simulink model "vehiclemodel"  (R2019a)
settings: Solver=VariableStepAuto  StartTime=0.0  StopTime=10.0  RelTol=1e-3
libraries: simulink x2, autolibshared x1
settings Model: Creator=L  LastModifiedBy=L

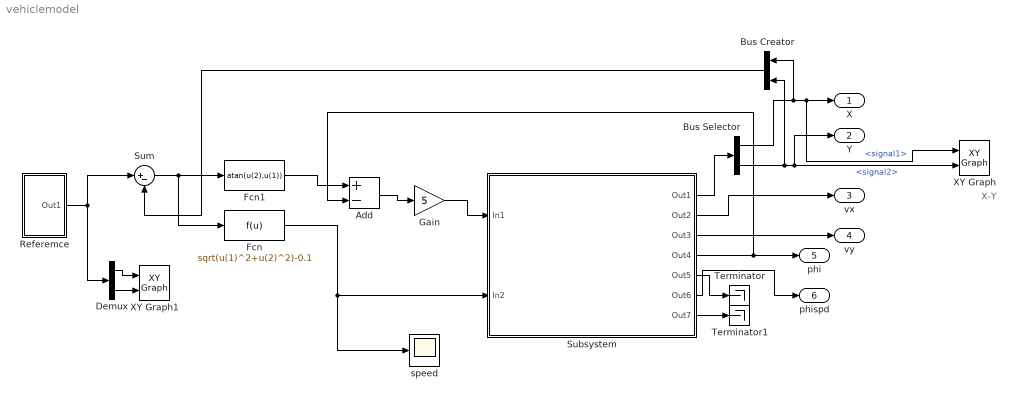
== system vehiclemodel ==
  note: X-Y
  Add : Sum  Inputs=+-
  Bus Creator : BusCreator  Inputs=2
  Bus Selector : BusSelector  OutputSignals=signal1,signal2
  Demux : Demux  Outputs=2
  Fcn : Fcn  Expr=sqrt(u(1)^2+u(2)^2)-0.1
  Fcn1 : Fcn  Expr=atan(u(2),u(1))
  Gain : Gain  Gain=5
  Referemce : Subsystem
  Subsystem : Subsystem
  Sum : Sum  Inputs=|+-
  Terminator : Terminator
  Terminator1 : Terminator
  XY Graph : simulink/Sinks/XY Graph  xmin=-1  xmax=1  ymin=-1  ymax=1  st=-1
  XY Graph1 : simulink/Sinks/XY Graph  xmin=-1  xmax=1  ymin=-1  ymax=1  st=-1
  speed : Scope
  X : Outport
  Y : Outport  Port=2
  vx : Outport  Port=3
  vy : Outport  Port=4
  phi : Outport  Port=5
  phispd : Outport  Port=6
  wires:
  Bus Selector/1 -> Bus Creator/1, XY Graph/1, X/1  "<signal1>"
  Bus Selector/2 -> Bus Creator/2, XY Graph/2, Y/1  "<signal2>"
  Demux/1 -> XY Graph1/1
  Demux/2 -> XY Graph1/2
  Referemce/1(Out1) -> Sum/1, Demux/1
  Bus Creator/1 -> Sum/2
  Sum/1 -> Fcn/1, Fcn1/1
  Fcn/1 -> Subsystem/2(In2), speed/1
  Fcn1/1 -> Add/1
  Add/1 -> Gain/1
  Subsystem/4(Out4) -> Add/2, phi/1
  Gain/1 -> Subsystem/1(In1)
  Subsystem/1(Out1) -> Bus Selector/1
  Subsystem/2(Out2) -> vx/1
  Subsystem/3(Out3) -> vy/1
  Subsystem/5(Out5) -> Terminator/1
  Subsystem/6(Out6) -> phispd/1
  Subsystem/7(Out7) -> Terminator1/1

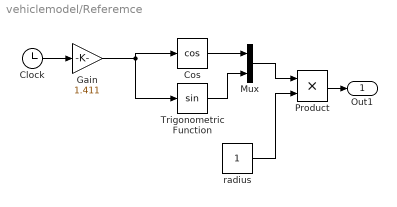
== system vehiclemodel/Referemce ==
  Clock : Clock
  Cos : Trigonometry  Operator=cos
  Gain : Gain  Gain=1.411
  Mux : Mux  Inputs=2
  Product : Product
  Trigonometric Function : Trigonometry
  radius : Constant
  Out1 : Outport
  wires:
  radius/1 -> Product/2
  Mux/1 -> Product/1
  Clock/1 -> Gain/1
  Gain/1 -> Cos/1, Trigonometric Function/1
  Trigonometric Function/1 -> Mux/2
  Cos/1 -> Mux/1
  Product/1 -> Out1/1

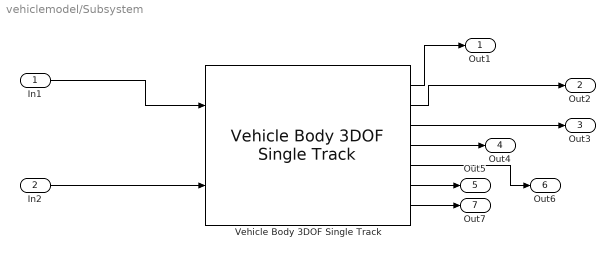
== system vehiclemodel/Subsystem ==
  In1 : Inport
  In2 : Inport  Port=2
  Vehicle Body 3DOF Single Track : autolibshared/Vehicle Body 3DOF Single Track  trackMode=Single (bicycle)  inputMode=External longitudinal velocity  frontSteerMode=on  rearSteerMode=off  windMode=off  muMode=off  extFMode=off  extMMode=off  extXo=off  extpsio=off  extxdoto=off  extro=off  extYo=off  extTamb=off  extydoto=off  aMode=2  NF=2  NR=2  m=2000  a=1.4  b=1.6  h=0.35  X_o=0  xdot_o=0  CalphaMode=off  sigmaMode=on  d=0  w=[1.4,1.4]  Cy_f=12e3  Cy_r=11e3  sigma_f=.1  sigma_r=.1  alpha_f_brk=[-.1 .1]  Cy_f_data=[-9e3 9e3]  alpha_r_brk=[-.1 .1]  Cy_r_data=[-9e3 9e3]  Y_o=0  ydot_o=0  Izz=4000  psi_o=0  r_o=0  Af=2  Cd=.3  Cl=.1  Cpm=.1  beta_w=[0:0.01:0.3]  Cs=[0:0.03:0.9]  Cym=[0:0.01:0.3]  Pabs=101325  Tair=273  g=9.81  mu=1  xdot_tol=.01  Fznom=5000  Fxtire_sat=7e4  Fytire_sat=7e4  longOff=0  latOff=0  vertOff=0  wrapAng=off  mask(Vehicle Body 3DOF Lateral){}
      settings: SourceProductName=Powertrain Blockset  SourceProductBaseCode=PW
  Out1 : Outport
  Out2 : Outport  Port=2
  Out3 : Outport  Port=3
  Out4 : Outport  Port=4
  Out5 : Outport  Port=5
  Out6 : Outport  Port=6
  Out7 : Outport  Port=7
  wires:
  Vehicle Body 3DOF Single Track/7 -> Out7/1
  Vehicle Body 3DOF Single Track/2 -> Out2/1
  Vehicle Body 3DOF Single Track/3 -> Out3/1
  Vehicle Body 3DOF Single Track/1 -> Out1/1
  In1/1 -> Vehicle Body 3DOF Single Track/1
  Vehicle Body 3DOF Single Track/6 -> Out5/1
  In2/1 -> Vehicle Body 3DOF Single Track/2
  Vehicle Body 3DOF Single Track/4 -> Out4/1
  Vehicle Body 3DOF Single Track/5 -> Out6/1
